simulink model "Q4cxLZuTCMuWW395RD0XXuXlqaU7t1KG2CoRlg85"  (R2020a)
settings: Solver=ode45  StartTime=0.0  StopTime=20  MaxStep=0.1  RelTol=1e-2  EnableMultiTasking=on
undefined symbols (not defined in the file or in its folder): ln, VETERR
libraries: simulink x3
settings Model: Creator=Andrey  LastModifiedBy=Tamer
settings SolverCC: AlgebraicLoopSolver=LineSearch
settings DataIOCC: LimitDataPoints=on  SaveFormat=Array  SignalLoggingSaveFormat=ModelDataLogs  ReturnWorkspaceOutputs=off
settings OptimizationCC: InitFltsAndDblsToZero=on  EfficientMapNaN2IntZero=off  LifeSpan=inf
settings DebuggingCC: SaveWithParameterizedLinksMsg=none  UnderspecifiedInitializationDetection=Classic  MergeDetectMultiDrivingBlocksExec=none  SignalResolutionControl=TryResolveAllWithWarning  MaxConsecutiveZCsMsg=none  SolverPrmCheckMsg=warning  MultiTaskDSMMsg=warning  MultiTaskCondExecSysMsg=none  FcnCallInpInsideContextMsg=warning  StateNameClashWarn=warning  SFUnexpectedBacktrackingDiag=warning  SFNoUnconditionalDefaultTransitionDiag=warning  SFExecutionAtInitializationDiag=none  ArithmeticOperatorsInVariantConditions=warning
settings HardwareCC: ProdBitPerPointer=32  ProdBitPerSizeT=32  ProdBitPerPtrDiffT=32  ProdLargestAtomicFloat=None  ProdIntDivRoundTo=Undefined  ProdEndianess=Unspecified  ProdWordSize=32  ProdHWDeviceType=32-bit Generic  TargetBitPerPointer=64  TargetBitPerSizeT=64  TargetBitPerPtrDiffT=64  TargetLongLongMode=on  TargetIntDivRoundTo=Zero  TargetEndianess=LittleEndian  TargetWordSize=64  TargetHWDeviceType=MATLAB Host  ProdEqTarget=off
settings ModelReferenceCC: PropagateSignalLabelsOutOfModel=off
settings SFSimCC: SimUseLocalCustomCode=off  CustomCodeUndefinedFunction=UseInterfaceOnly
settings RTWCC: RTWUseLocalCustomCode=off
settings CodeAppCC: MaxIdLength=128
settings GRTTargetCC: TargetLangStandard=C89/C90 (ANSI)  CombineOutputUpdateFcns=off  GRTInterface=on
settings ConfigComp: CovMetricSettings=dw  CovHtmlReporting=on  CovSaveCumulativeToWorkspaceVar=on  CovSaveSingleToWorkspaceVar=on  CovExternalEMLEnable=off

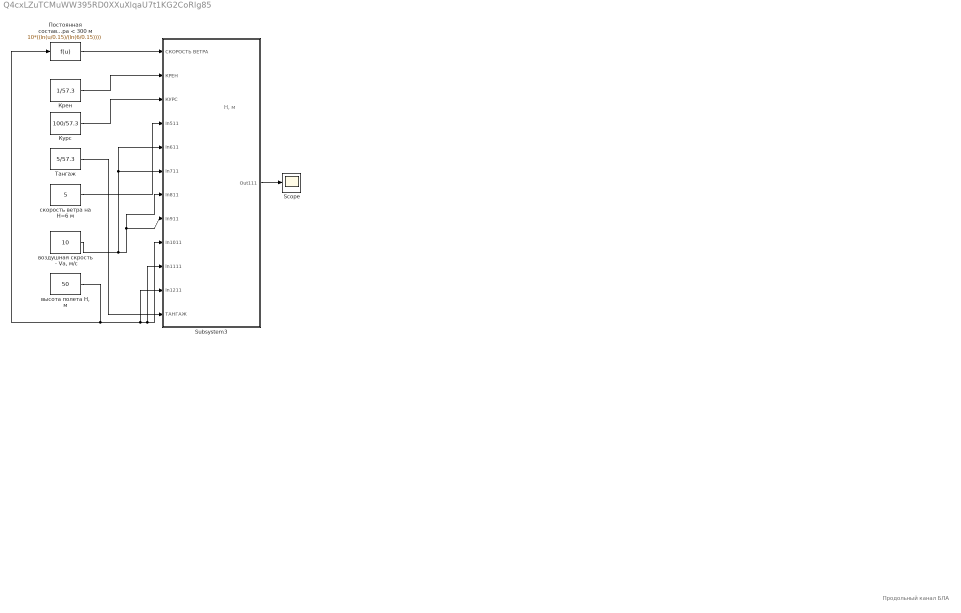
== system Q4cxLZuTCMuWW395RD0XXuXlqaU7t1KG2CoRlg85 ==
  note: Н, м
  note: Продольный канал БЛА
  "    Постоянная составляющая скорости ветра < 300 м" : Fcn  Expr=10*((ln(u/0.15)/(ln(6/0.15))))
  Scope : Scope
  Subsystem3 : Subsystem
  "Крен " : Constant  Value=1/57.3
  Курс : Constant  Value=100/57.3
  Тангаж : Constant  Value=5/57.3
  "воздушная скрость  - Vа, м/с" : Constant  Value=10
  "высота полета Н, м " : Constant  Value=50
  "скорость ветра на Н=6 м " : Constant  Value=5
  wires:
  Subsystem3/1(Out111) -> Scope/1
  "    Постоянная составляющая скорости ветра < 300 м"/1 -> Subsystem3/1("СКОРОСТЬ ВЕТРА ")
  "Крен "/1 -> Subsystem3/2(КРЕН)
  Курс/1 -> Subsystem3/3("КУРС ")
  "скорость ветра на Н=6 м "/1 -> Subsystem3/4(In511)
  "высота полета Н, м "/1 -> Subsystem3/9(In1011), Subsystem3/10(ln1111), Subsystem3/11(In1211), "    Постоянная составляющая скорости ветра < 300 м"/1
  "воздушная скрость  - Vа, м/с"/1 -> Subsystem3/5(In611), Subsystem3/6(In711), Subsystem3/7(In811), Subsystem3/8(In911)
  Тангаж/1 -> Subsystem3/12("ТАНГАЖ ")

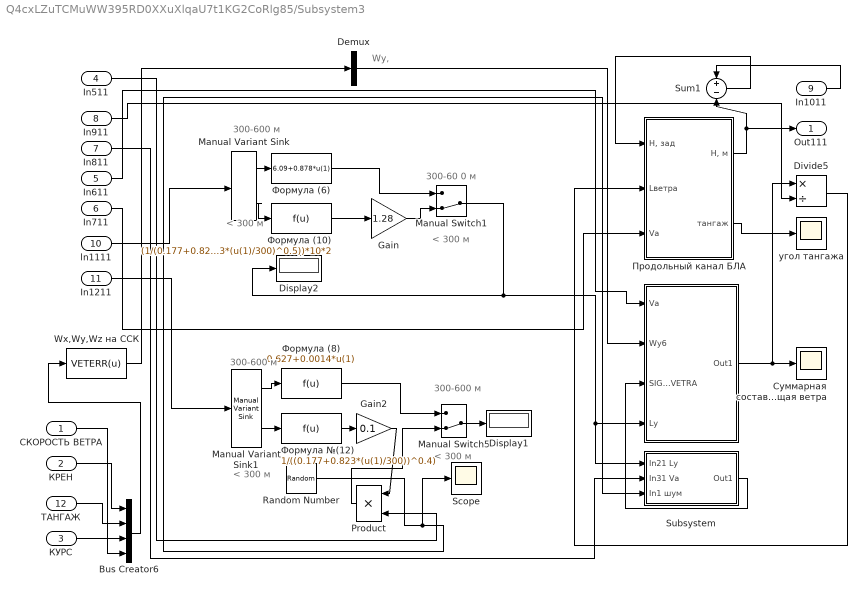
== system Q4cxLZuTCMuWW395RD0XXuXlqaU7t1KG2CoRlg85/Subsystem3 ==
  note: Wy,
  note: < 300 м
  note: < 300 м
  note: 300-600 м
  note: < 300 м
  note: 300-60 0 м
  note: 300-600 м
  note: < 300 м
  note: 300-600 м
  "СКОРОСТЬ ВЕТРА " : Inport
  КРЕН : Inport  Port=2
  "КУРС " : Inport  Port=3
  In511 : Inport  Port=4
  In611 : Inport  Port=5
  In711 : Inport  Port=6
  In811 : Inport  Port=7
  In911 : Inport  Port=8
  In1011 : Inport  Port=9
  ln1111 : Inport  Port=10
  In1211 : Inport  Port=11
  "ТАНГАЖ " : Inport  Port=12
  " " : Subsystem
  " Wх,Wy,Wz на ССК" : MATLABFcn  MATLABFcn=VETERR(u)  OutputDimensions=3
  Bus Creator6 : BusCreator  Inputs=4
  Demux : Demux  Outputs=3
  Display1 : Display
  Display2 : Display
  Divide5 : Product  Inputs=*/
  Gain : Gain  Gain=1.28
  Gain2 : Gain  Gain=0.1
  Manual Variant Sink : simulink/Signal Routing/Manual Variant Sink  NumChoices=2  LabelModeActiveChoice=V_2
  Manual Variant Sink1 : simulink/Signal Routing/Manual Variant Sink  NumChoices=2  LabelModeActiveChoice=V_2
  Manual Switch1 : ManualSwitch  CurrentSetting=0
  Manual Switch5 : ManualSwitch  CurrentSetting=0
  Product : Product
  Random Number : RandomNumber  Variance=0.79*0.79  Seed=984387543544345  SampleTime=0.1
  Scope : Scope
  Subsystem : Subsystem
  Sum1 : Sum  Inputs=+-
  Продольный канал БЛА : Subsystem
  Суммарная составляющая ветра : Scope
  Формула (10) : Fcn  Expr=(1/(0.177+0.823*(u(1)/300)^0.5))*10*2
  Формула (6) : Fcn  Expr=6.09+0.878*u(1)
  Формула (8) : Fcn  Expr=0.627+0.0014*u(1)
  Формула №(12) : Fcn  Expr=1/((0.177+0.823*(u(1)/300))^0.4)
  "угол тангажа " : Scope
  Out111 : Outport  VectorParamsAs1DForOutWhenUnconnected=off
  wires:
  In511/1 -> Product/2
  Divide5/1 -> Продольный канал БЛА/2(Lветра)
  Random Number/1 -> Subsystem/3("In1 шум "), Scope/1
  Manual Switch1/1 -> Display2/1, Subsystem/1("In21 Ly "), " "/4(Ly)
  Формула (10)/1 -> Gain/1
  Manual Variant Sink/1 -> Формула (6)/1
  Sum1/1 -> Продольный канал БЛА/1("Н, зад")
  Продольный канал БЛА/1("Н, м ") -> Sum1/2, Out111/1
  Demux/2 -> " "/2(Wy6)
  " Wх,Wy,Wz на ССК"/1 -> Demux/1
  Subsystem/1(Out1) -> " "/3("SIGMA VETRA ")
  Manual Variant Sink/2 -> Формула (10)/1
  " "/1(Out1) -> Суммарная составляющая ветра/1, Divide5/1
  КРЕН/1 -> Bus Creator6/1
  Bus Creator6/1 -> " Wх,Wy,Wz на ССК"/1
  "КУРС "/1 -> Bus Creator6/3
  In911/1 -> Divide5/2
  In811/1 -> Subsystem/2(In31 Va)
  In1211/1 -> Manual Variant Sink1/1
  In1011/1 -> Sum1/1
  "СКОРОСТЬ ВЕТРА "/1 -> Bus Creator6/4
  In611/1 -> " "/1(Va)
  In711/1 -> Продольный канал БЛА/3(Va)
  ln1111/1 -> Manual Variant Sink/1
  Gain2/1 -> Product/1
  Manual Variant Sink1/1 -> Формула (8)/1
  Формула (8)/1 -> Manual Switch5/1
  Формула №(12)/1 -> Gain2/1
  Product/1 -> Manual Switch5/2
  Manual Variant Sink1/2 -> Формула №(12)/1
  Manual Switch5/1 -> Display1/1
  Формула (6)/1 -> Manual Switch1/1
  Gain/1 -> Manual Switch1/2
  Продольный канал БЛА/2("тангаж ") -> "угол тангажа "/1
  "ТАНГАЖ "/1 -> Bus Creator6/2

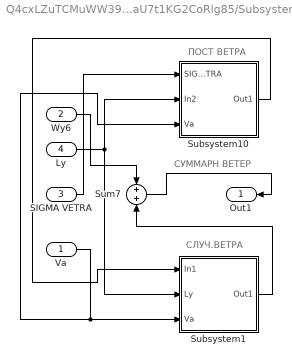
== system Q4cxLZuTCMuWW395RD0XXuXlqaU7t1KG2CoRlg85/Subsystem3/  ==
  note: СУММАРН ВЕТЕР
  note: ПОСТ ВЕТРА
  note: СЛУЧ.ВЕТРА
  Va : Inport
  Wy6 : Inport  Port=2
  "SIGMA VETRA " : Inport  Port=3
  Ly : Inport  Port=4
  Subsystem1 : Subsystem
  "Subsystem10 " : Subsystem
  Sum7 : Sum
  Out1 : Outport  VectorParamsAs1DForOutWhenUnconnected=off
  wires:
  Wy6/1 -> Sum7/1
  Sum7/1 -> Out1/1
  Ly/1 -> Subsystem1/2(Ly), "Subsystem10 "/2(In2)
  "SIGMA VETRA "/1 -> "Subsystem10 "/1(SIGMA VETRA)
  "Subsystem10 "/1(Out1) -> Subsystem1/1(In1)
  Va/1 -> "Subsystem10 "/3("Va "), Subsystem1/3(Va)
  Subsystem1/1(Out1) -> Sum7/2

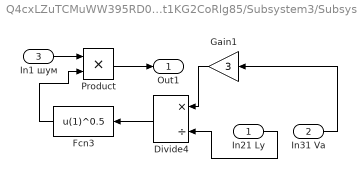
== system Q4cxLZuTCMuWW395RD0XXuXlqaU7t1KG2CoRlg85/Subsystem3/Subsystem ==
  "In21 Ly " : Inport
  In31 Va : Inport  Port=2
  "In1 шум " : Inport  Port=3
  Divide4 : Product  Inputs=*/
  Fcn3 : Fcn  Expr=u(1)^0.5
  Gain1 : Gain  Gain=3
  Product : Product
  Out1 : Outport  VectorParamsAs1DForOutWhenUnconnected=off
  wires:
  In31 Va/1 -> Gain1/1
  Gain1/1 -> Divide4/1
  Divide4/1 -> Fcn3/1
  "In21 Ly "/1 -> Divide4/2
  Fcn3/1 -> Product/2
  Product/1 -> Out1/1
  "In1 шум "/1 -> Product/1

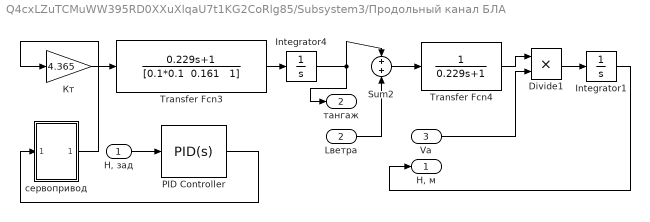
== system Q4cxLZuTCMuWW395RD0XXuXlqaU7t1KG2CoRlg85/Subsystem3/Продольный канал БЛА ==
  "Н, зад" : Inport
  Lветра : Inport  Port=2
  Va : Inport  Port=3
  Divide1 : Product  Inputs=**
  Integrator1 : Integrator
  Integrator4 : Integrator
  PID Controller : simulink/Continuous/PID Controller  Controller=PID  Form=Parallel  TimeDomain=Continuous-time  UseExternalTs=off  SampleTime=-1  IntegratorMethod=Forward Euler  FilterMethod=Forward Euler  ControllerParametersSource=internal  P=0.00618279235491519  I=0.00618*0.5/3  D=0.00618  UseFilter=on  N=1/0.00618  TunerSelectOption=Transfer Function Based (PID Tuner App)  InitialConditionSource=internal  InitialConditionForIntegrator=0  InitialConditionForFilter=0  DifferentiatorICPrevScaledInput=0  ExternalReset=none  TrackingMode=off  Kt=1  LimitOutput=off  UpperSaturationLimit=inf  LowerSaturationLimit=-inf  LinearizeAsGain=on  AntiWindupMode=none  Kb=1  POutMin=[]  POutMax=[]  IOutMin=[]  IOutMax=[]  DOutMin=[]  DOutMax=[]  NOutMin=[]  NOutMax=[]  SumOutMin=[]  SumOutMax=[]  SaturationOutMin=[]  SaturationOutMax=[]  PParamMin=[]  PParamMax=[]  IParamMin=[]  IParamMax=[]  DParamMin=[]  DParamMax=[]  NParamMin=[]  NParamMax=[]  KbParamMin=[]  KbParamMax=[]  KtParamMin=[]  KtParamMax=[]  KbOutMin=[]  KbOutMax=[]  KtOutMin=[]  KtOutMax=[]  IntegratorOutMin=[]  IntegratorOutMax=[]  FilterOutMin=[]  FilterOutMax=[]  SumI1OutMin=[]  SumI1OutMax=[]  SumI2OutMin=[]  SumI2OutMax=[]  SumI3OutMin=[]  SumI3OutMax=[]  SumI4OutMin=[]  SumI4OutMax=[]  SumDOutMin=[]  SumDOutMax=[]  DifferentiatorOutMin=[]  DifferentiatorOutMax=[]  FilterDiffOutCoefMin=[]  FilterDiffOutCoefMax=[]  ReciprocalOutMin=[]  ReciprocalOutMax=[]  SumDenOutMin=[]  SumDenOutMax=[]  SumNumOutMin=[]  SumNumOutMax=[]  DivideOutMin=[]  DivideOutMax=[]  UdiffTsProdOutMin=[]  UdiffTsProdOutMax=[]  NTsProdOutMin=[]  NTsProdOutMax=[]  UintegralTsProdOutMin=[]  UintegralTsProdOutMax=[]  UngainTsProdOutMin=[]  UngainTsProdOutMax=[]  IntegratorContinuousStateAttributes=''  IntegratorStateMustResolveToSignalObject=off  IntegratorRTWStateStorageClass=Auto  FilterContinuousStateAttributes=''  FilterStateMustResolveToSignalObject=off  FilterRTWStateStorageClass=Auto  ParallelPVariant=InternalParameters  IdealPVariant=Disabled  IVariant=InternalParameters  DVariant=InternalParameters  IntegratorVariant=Continuous  SatVariant=Disabled  AWVariant=Passthrough  PCopyVariant=Disabled  TRVariant=Disabled  FdbkBlocksVariant=Forward  IdealPFdbkVariant=Disabled  SatFdbkVariant=Disabled  DerivativeFilterVariant=ContFilter  NVariant=InternalParameters  NCopyVariant=Disabled  FilterICVariant=InternalICsFilter  IntegratorICVariant=InternalICs  ExternalResetVariant=Disabled  TRSumVariant=Passthrough  SumFdbkVariant=Disabled  SumVariant=Sum_PID  TsampFilterVariant=InternalTs  TsampNgainVariant=Passthrough  TsampIntegralVariant=Passthrough
  Sum2 : Sum
  Transfer Fcn3 : TransferFcn  Numerator="[0.229  1]"  Denominator="[0.1*0.1  0.161   1]"
  Transfer Fcn4 : TransferFcn  Denominator="[0.229  1]"
  "Кт " : Gain  Gain=4.365
  сервопривод : Subsystem
  "Н, м " : Outport  VectorParamsAs1DForOutWhenUnconnected=off
  "тангаж " : Outport  Port=2  VectorParamsAs1DForOutWhenUnconnected=off
  wires:
  Transfer Fcn3/1 -> Integrator4/1
  Integrator4/1 -> "тангаж "/1, Sum2/1
  "Н, зад"/1 -> PID Controller/1
  сервопривод/1(Out1) -> "Кт "/1
  Integrator1/1 -> "Н, м "/1
  Transfer Fcn4/1 -> Divide1/1
  PID Controller/1 -> сервопривод/1(In1)
  "Кт "/1 -> Transfer Fcn3/1
  Divide1/1 -> Integrator1/1
  Sum2/1 -> Transfer Fcn4/1
  Lветра/1 -> Sum2/2
  Va/1 -> Divide1/2

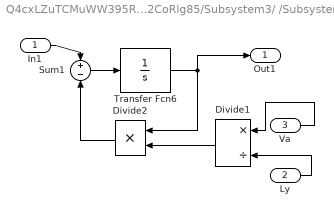
== system Q4cxLZuTCMuWW395RD0XXuXlqaU7t1KG2CoRlg85/Subsystem3/ /Subsystem1 ==
  In1 : Inport
  Ly : Inport  Port=2
  Va : Inport  Port=3
  Divide1 : Product  Inputs=*/
  Divide2 : Product  Inputs=**
  Sum1 : Sum  Inputs=+-
  Transfer Fcn6 : TransferFcn  Denominator="[1  0]"
  Out1 : Outport  VectorParamsAs1DForOutWhenUnconnected=off
  wires:
  Va/1 -> Divide1/1
  Divide1/1 -> Divide2/2
  In1/1 -> Sum1/1
  Transfer Fcn6/1 -> Out1/1, Divide2/1
  Divide2/1 -> Sum1/2
  Ly/1 -> Divide1/2
  Sum1/1 -> Transfer Fcn6/1

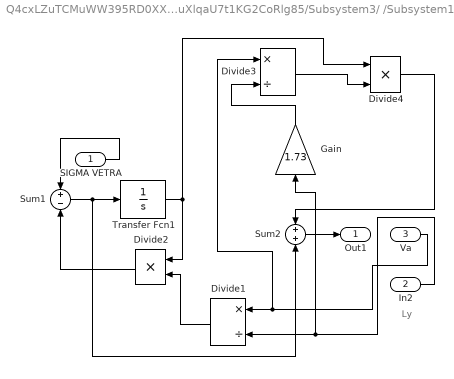
== system Q4cxLZuTCMuWW395RD0XXuXlqaU7t1KG2CoRlg85/Subsystem3/ /Subsystem10  ==
  note: Ly
  SIGMA VETRA : Inport
  In2 : Inport  Port=2
  "Va " : Inport  Port=3
  Divide1 : Product  Inputs=*/
  Divide2 : Product  Inputs=**
  Divide3 : Product  Inputs=*/
  Divide4 : Product  Inputs=**
  Gain : Gain  Gain=1.73
  Sum1 : Sum  Inputs=+-
  Sum2 : Sum
  Transfer Fcn1 : TransferFcn  Denominator="[1  0]"
  Out1 : Outport  VectorParamsAs1DForOutWhenUnconnected=off
  wires:
  Divide1/1 -> Divide2/2
  SIGMA VETRA/1 -> Sum1/1
  Divide2/1 -> Sum1/2
  In2/1 -> Divide1/2, Gain/1
  Transfer Fcn1/1 -> Divide2/1, Divide4/1
  Sum2/1 -> Out1/1
  "Va "/1 -> Divide3/1, Divide1/1
  Sum1/1 -> Sum2/2, Transfer Fcn1/1
  Divide4/1 -> Sum2/1
  Divide3/1 -> Divide4/2
  Gain/1 -> Divide3/2

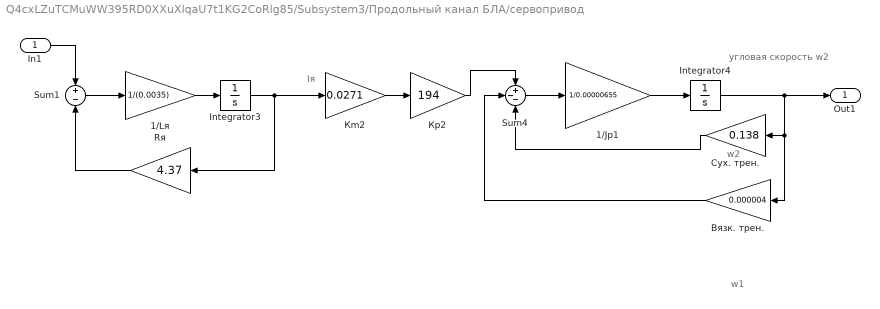
== system Q4cxLZuTCMuWW395RD0XXuXlqaU7t1KG2CoRlg85/Subsystem3/Продольный канал БЛА/сервопривод ==
  note: Iя
  note: w1
  note: w2
  note: угловая
      | скорость w2
  In1 : Inport
  "           Вязк. трен. " : Gain  Gain=0.000004
  "           Сух. трен. " : Gain  Gain=0.138
  1/Jp1 : Gain  Gain=1/0.00000655
  "1/Lя " : Gain  Gain=1/(0.0035)
  Integrator3 : Integrator
  Integrator4 : Integrator
  Rя : Gain  Gain=4.37
  Sum1 : Sum  Inputs=+-
  Sum4 : Sum  Inputs=+--
  Кm2 : Gain  Gain=0.0271
  Кp2 : Gain  Gain=194
  Out1 : Outport  VectorParamsAs1DForOutWhenUnconnected=off
  wires:
  1/Jp1/1 -> Integrator4/1
  "           Сух. трен. "/1 -> Sum4/3
  Sum4/1 -> 1/Jp1/1
  Кp2/1 -> Sum4/1
  Integrator3/1 -> Кm2/1, Rя/1
  "1/Lя "/1 -> Integrator3/1
  Sum1/1 -> "1/Lя "/1
  Кm2/1 -> Кp2/1
  "           Вязк. трен. "/1 -> Sum4/2
  Integrator4/1 -> Out1/1, "           Вязк. трен. "/1, "           Сух. трен. "/1
  Rя/1 -> Sum1/2
  In1/1 -> Sum1/1
